simulink model "Three_phase_vsi_without_pwm_technique"  (R2014a)
settings: Solver=ode23t  StartTime=0.0  StopTime=1  MaxStep=1e-6  RelTol=1e-3
libraries: powerlib x17, powerlib_meascontrol x2
settings Model: Creator=singa  LastModifiedBy=singa

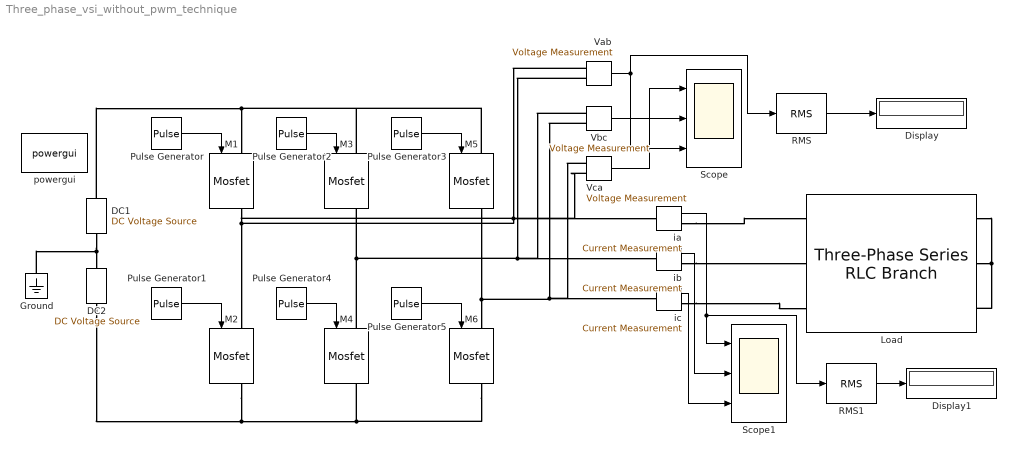
== system Three_phase_vsi_without_pwm_technique ==
  DC1 : powerlib/Electrical Sources/DC Voltage Source  Amplitude=50  Measurements=None
  DC2 : powerlib/Electrical Sources/DC Voltage Source  Amplitude=50  Measurements=None
  Display : Display
  Display1 : Display
  Ground : powerlib/Elements/Ground  LConnTagsString=a
  Load : powerlib/Elements/Three-Phase Series RLC Branch  LConnTagsString=A|B|C  RConnTagsString=A|B|C  BranchType=RL  Resistance=1  Inductance=1e-2  Capacitance=1e-6  Measurements=None
  M{1..6} (6 alike) : powerlib/Power Electronics/Mosfet  Ron=0.1  Lon=0  Rd=0.01  Vfd=0  IC=0  Rs=1e5  Cs=inf  Measurements=on
  Pulse Generator : DiscretePulseGenerator  PulseType=Time based  Period=0.02  PulseWidth=50
  Pulse Generator1 : DiscretePulseGenerator  PulseType=Time based  Period=0.02  PulseWidth=50  PhaseDelay=0.01
  Pulse Generator2 : DiscretePulseGenerator  PulseType=Time based  Period=0.02  PulseWidth=50  PhaseDelay=0.02/3
  Pulse Generator3 : DiscretePulseGenerator  PulseType=Time based  Period=0.02  PulseWidth=50  PhaseDelay=0.04/3
  Pulse Generator4 : DiscretePulseGenerator  PulseType=Time based  Period=0.02  PulseWidth=50  PhaseDelay=0.01+0.02/3
  Pulse Generator5 : DiscretePulseGenerator  PulseType=Time based  Period=0.02  PulseWidth=50  PhaseDelay=0.01+0.04/3
  RMS : powerlib_meascontrol/Measurements/RMS  TrueRMS=on  Freq=50  RMSInit=0  Ts=0
  RMS1 : powerlib_meascontrol/Measurements/RMS  TrueRMS=on  Freq=50  RMSInit=0  Ts=0
  Scope : Scope  NumInputPorts=3
      settings: YMin=-5~-5~-5  YMax=5~5~5  SampleInput=on  SampleTime=1e-6
  Scope1 : Scope  NumInputPorts=3
      settings: YMin=-5~-5~-5  YMax=5~5~5  SampleInput=on  SampleTime=1e-6
  Vab : powerlib/Measurements/Voltage Measurement  PhasorSimulation=off  OutputType=Complex  PSBequivalent=0
  Vbc : powerlib/Measurements/Voltage Measurement  PhasorSimulation=off  OutputType=Complex  PSBequivalent=0
  Vca : powerlib/Measurements/Voltage Measurement  PhasorSimulation=off  OutputType=Complex  PSBequivalent=0
  ia : powerlib/Measurements/Current Measurement  PhasorSimulation=off  OutputType=Complex  PSBequivalent=0
  ib : powerlib/Measurements/Current Measurement  PhasorSimulation=off  OutputType=Complex  PSBequivalent=0
  ic : powerlib/Measurements/Current Measurement  PhasorSimulation=off  OutputType=Complex  PSBequivalent=0
  powergui : powerlib/powergui  Priority=1  SimulationMode=Continuous  SolverType=Tustin  SampleTime=50e-6  frequency=60  SPID=off  DisableSnubberDevices=off  DisableRonSwitches=off  DisableVfSwitches=off  SwTol=0  Interpol=off  DisplayEquations=off  Ts=0  methode=off  frequencyindice=0  Pbase=100e6  ErrMax=1e-4  Iterations=50  UnitsV=kV  UnitsW=MW  FunctionMessages=off  echomessages=off  HookPort=off  EnableUseOfTLC=off  x0status=blocks  RestoreLinks=warning  ResistiveCurrentMeasurement=off  Frange=[0:2:500]  Ylog=off  Xlog=on  ShowGrid=off  save=off  variable=ZData  structure=ScopeData  ZoomFFT=off  StartTime=0.8  cycles=2  DisplayStyle=4  fundamental=50  FreqAxis=on  MaxFrequency=2500  frequencyindicesteady=1  RmsSteady=1  display=off
  wires:
  Pulse Generator/1 -> M1/1
  Pulse Generator1/1 -> M2/1
  Pulse Generator2/1 -> M3/1
  Pulse Generator3/1 -> M5/1
  Pulse Generator4/1 -> M4/1
  Pulse Generator5/1 -> M6/1
  Vab/1 -> Scope/3, RMS/1
  Vbc/1 -> Scope/2
  Vca/1 -> Scope/1
  ia/1 -> Scope1/1, RMS1/1
  ib/1 -> Scope1/2
  ic/1 -> Scope1/3
  RMS/1 -> Display/1
  RMS1/1 -> Display1/1
  connections:
  DC1/LConn1 -- Ground/LConn1 -- DC2/RConn1
  DC1/RConn1 -- M5/LConn1 -- M3/LConn1 -- M1/LConn1
  M1/RConn1 -- Vca/LConn2 -- ia/LConn1 -- Vab/LConn1 -- M2/LConn1
  M4/LConn1 -- M3/RConn1 -- Vab/LConn2 -- Vbc/LConn1 -- ib/LConn1
  M2/RConn1 -- M6/RConn1 -- M4/RConn1 -- DC2/LConn1
  M5/RConn1 -- Vbc/LConn2 -- Vca/LConn1 -- ic/LConn1 -- M6/LConn1
  Load/RConn1 -- Load/RConn3 -- Load/RConn2
  ia/RConn1 -- Load/LConn1
  ib/RConn1 -- Load/LConn2
  ic/RConn1 -- Load/LConn3
